simulink model "problem2Simulink"  (R2023a)
settings: Solver=VariableStepAuto  StartTime=0.0  StopTime=50  RelTol=1e-3
undefined symbols (not defined in the file): a1, A1, A2, a2, g, K
settings Model: Creator=may8  LastModifiedBy=qnmdgpqs

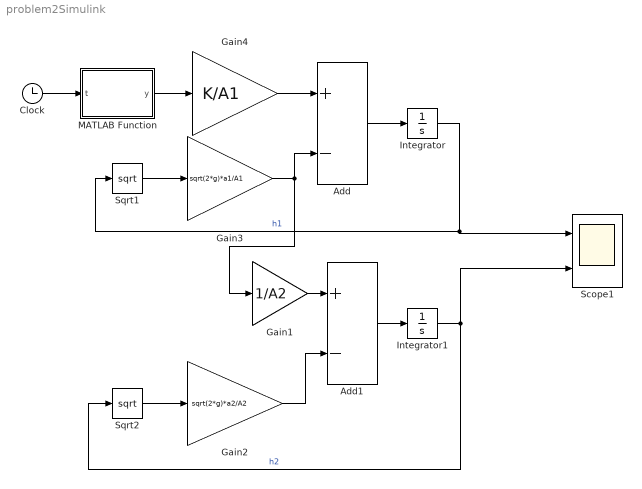
== system problem2Simulink ==
  Add : Sum  Inputs=+-
  Add1 : Sum  Inputs=+-
  Clock : Clock
  Gain1 : Gain  Gain=1/A2
  Gain2 : Gain  Gain=sqrt(2*g)*a2/A2
  Gain3 : Gain  Gain=sqrt(2*g)*a1/A1
  Gain4 : Gain  Gain=K/A1
  Integrator : Integrator  InitialCondition=1
  Integrator1 : Integrator
  MATLAB Function : MATLAB Function  TreatAsAtomicUnit=on
  Scope1 : Scope  NumInputPorts=2
  Sqrt1 : Sqrt
  Sqrt2 : Sqrt
  wires:
  Gain3/1 -> Gain1/1, Add/2
  Gain2/1 -> Add1/2
  Sqrt1/1 -> Gain3/1
  Add/1 -> Integrator/1
  Sqrt2/1 -> Gain2/1
  Add1/1 -> Integrator1/1
  Integrator/1 -> Scope1/1, Sqrt1/1  "h1"
  Integrator1/1 -> Sqrt2/1, Scope1/2  "h2"
  Gain1/1 -> Add1/1
  Clock/1 -> MATLAB Function/1(t)
  Gain4/1 -> Add/1
  MATLAB Function/1(y) -> Gain4/1

== matlab function problem2Simulink/MATLAB Function ==
  data: t input; y output
function y = fcn(t)
    y =  1 + 0.1*sin(t);
% y = u;
